simulink library "lib_decmp_Calib_tbm_sensor_x4"  (R2020a)
settings: Solver=VariableStepAuto  StartTime=0.0  StopTime=10.0  RelTol=1e-3
settings Model: Creator=Administrator  LastModifiedBy=Administrator

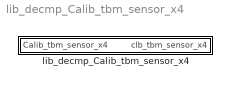
== system lib_decmp_Calib_tbm_sensor_x4 ==
  lib_decmp_Calib_tbm_sensor_x4 : Subsystem

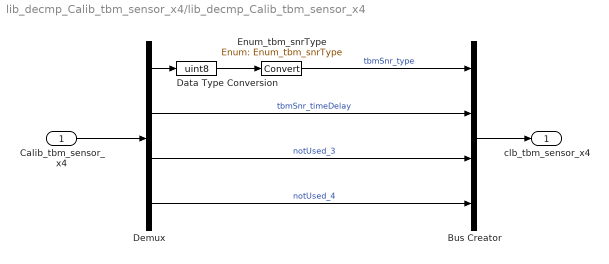
== system lib_decmp_Calib_tbm_sensor_x4/lib_decmp_Calib_tbm_sensor_x4 ==
  Calib_tbm_sensor_x4 : Inport  OutDataTypeStr=single  PortDimensions=4
  Bus Creator : BusCreator  Inputs=4
  Data Type Conversion : DataTypeConversion  OutDataTypeStr=uint8  RndMeth=Nearest
  Demux : Demux
  Enum_tbm_snrType : DataTypeConversion  OutDataTypeStr=Enum: Enum_tbm_snrType  RndMeth=Nearest
  clb_tbm_sensor_x4 : Outport  PortDimensions=4
  wires:
  Calib_tbm_sensor_x4/1 -> Demux/1
  Bus Creator/1 -> clb_tbm_sensor_x4/1
  Demux/1 -> Data Type Conversion/1
  Demux/3 -> Bus Creator/3  "notUsed_3"
  Demux/4 -> Bus Creator/4  "notUsed_4"
  Data Type Conversion/1 -> Enum_tbm_snrType/1
  Enum_tbm_snrType/1 -> Bus Creator/1  "tbmSnr_type"
  Demux/2 -> Bus Creator/2  "tbmSnr_timeDelay"
